simulink model "main_servo"  (R2019b)
settings: Solver=VariableStepAuto  StartTime=0.0  StopTime=60  MaxStep=0.01  RelTol=1e-3
undefined symbols (not defined in the file): __PRM__SERIALIZED__DATA__, SubsystemReferenceBlock
settings Model: Creator=toons  LastModifiedBy=toons

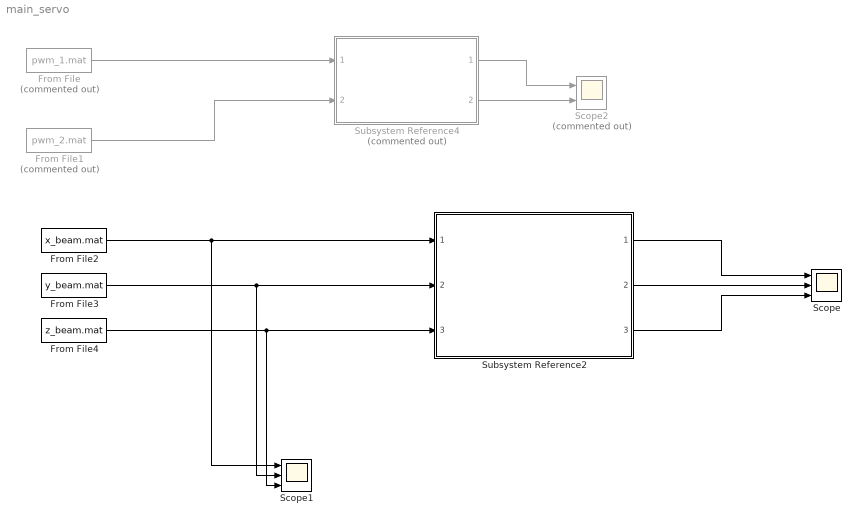
== system main_servo ==
  From File : FromFile  Commented=on  FileName=pwm_1.mat
  From File1 : FromFile  Commented=on  FileName=pwm_2.mat
  From File2 : FromFile  FileName=x_beam.mat
  From File3 : FromFile  FileName=y_beam.mat
  From File4 : FromFile  FileName=z_beam.mat
  Scope : Scope  NumInputPorts=3
  Scope1 : Scope  NumInputPorts=3
  Scope2 : Scope  Commented=on  NumInputPorts=2
  Subsystem Reference2 : Subsystem  BlockKeywords=__PRM__SERIALIZED__DATA__:SubsystemReferenceBlock  ReferencedSubsystem=Kalman_Filter
  Subsystem Reference4 : Subsystem  Commented=on  BlockKeywords=__PRM__SERIALIZED__DATA__:SubsystemReferenceBlock  ReferencedSubsystem=ServoSimulation
  wires:
  From File1/1 -> Subsystem Reference4/2
  From File/1 -> Subsystem Reference4/1
  Subsystem Reference4/1 -> Scope2/1
  Subsystem Reference4/2 -> Scope2/2
  From File3/1 -> Subsystem Reference2/2, Scope1/2
  From File2/1 -> Subsystem Reference2/1, Scope1/1
  From File4/1 -> Scope1/3, Subsystem Reference2/3
  Subsystem Reference2/2 -> Scope/2
  Subsystem Reference2/1 -> Scope/1
  Subsystem Reference2/3 -> Scope/3
